simulink model "EvitaParedes23"  (R2023b)
settings: Solver=FixedStepAuto  StartTime=0.0  StopTime=inf  RelTol=1e-3  EnableMultiTasking=on
libraries: arduinolib x11, simulink x4
settings Model: PacingRate=1.500000  ExtModeTrigDuration=2  Creator=manu_  LastModifiedBy=manu_
settings OptimizationCC: EnhancedBackFolding=on  PassReuseOutputArgsAs=Individual arguments  ZeroExternalMemoryAtStartup=off  ZeroInternalMemoryAtStartup=off  MaxStackSize=64  OptimizeBlockOrder=speed  DifferentSizesBufferReuse=on  OptimizationCustomize=off  EfficientTunableParamExpr=on
settings DebuggingCC: ParameterTunabilityLossMsg=error
settings HardwareCC: ProdBitPerInt=16  ProdBitPerPointer=16  ProdBitPerSizeT=16  ProdBitPerPtrDiffT=16  ProdLargestAtomicFloat=None  ProdWordSize=8  ProdHWDeviceType=Atmel->AVR  UseEmbeddedCoderFeatures=off  UseSimulinkCoderFeatures=off
settings SFSimCC: MATLABDynamicMemAlloc=off
settings RTWCC: Description=Embedded Coder  SystemTargetFile=ert.tlc  HardwareBoard=Arduino Mega 2560  TemplateMakefile=ert_default_tmf  Toolchain=Arduino AVR  BuildConfiguration=Faster Runs
settings CodeAppCC: ForceParamTrailComments=on  IgnoreCustomStorageClasses=off  OperatorAnnotations=on  SimulinkDataObjDesc=on  SFDataObjDesc=on  MangleLength=10  InsertBlockDesc=on
settings ERTTargetCC: SupportContinuousTime=on  SupportNonInlinedSFcns=on  SupportVariableSizeSignals=on  ExtModeTransport=3  ExtModeStaticAlloc=on  ExtModeAutomaticAllocSize=off  ExtModeStaticAllocSize=2048  ExtModeMexFile=ext_xcp  ExtModeIntrfLevel=Level2 - Open

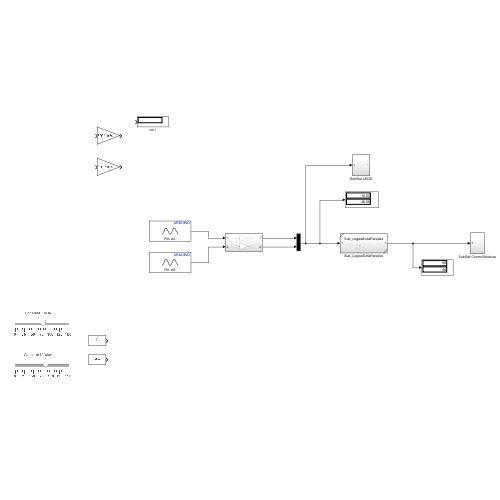
[thumbnail: Simulink's stored preview of the top-level diagram]
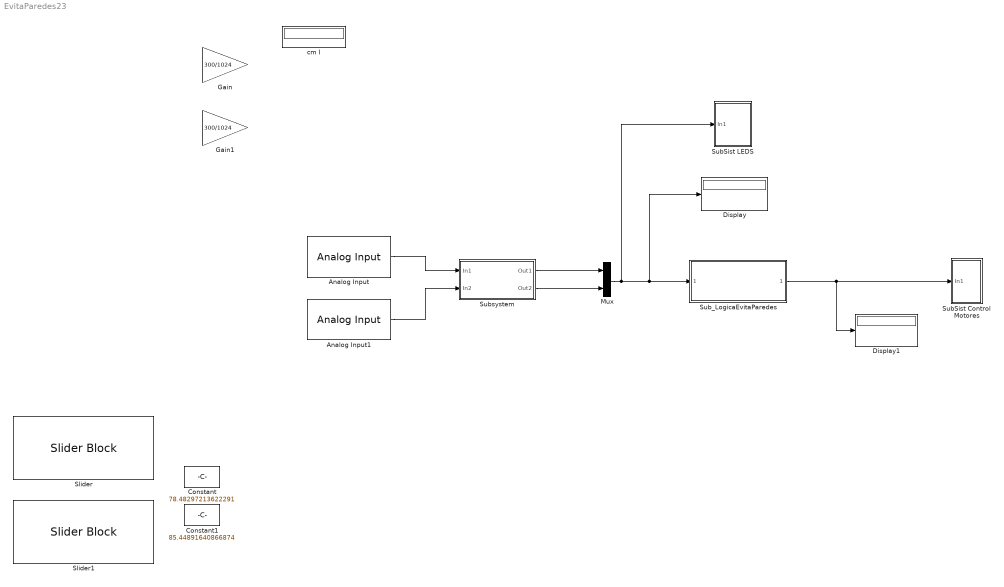
== system EvitaParedes23 ==
  Analog Input : arduinolib/Analog Input  pinNumber=4  ReadResultsOnly=off  ConversionTriggerSource=Software  ExternalTriggerType=uint32( 0 )  OutputDataType=uint16  EnableConversionCompleteNotify=off  EnableOuputStatus=off  SampleTime=-1  blockPlatform=arduino
  Analog Input1 : arduinolib/Analog Input  pinNumber=5  ReadResultsOnly=off  ConversionTriggerSource=Software  ExternalTriggerType=uint32( 0 )  OutputDataType=uint16  EnableConversionCompleteNotify=off  EnableOuputStatus=off  SampleTime=-1  blockPlatform=arduino
  Constant : Constant  Value=78.48297213622291
  Constant1 : Constant  Value=85.44891640866874
  Display : Display
  Display1 : Display
  Gain : Gain  Gain=300/1024
  Gain1 : Gain  Gain=300/1024
  Mux : Mux  Inputs=2
  Slider : SliderBlock  ScaleMax=150
  Slider1 : SliderBlock  ScaleMax=150
  SubSist Control Motores : Subsystem
  SubSist LEDS : Subsystem
  Sub_LogicaEvitaParedes : Subsystem  ReferencedSubsystem=Sub_LogicaEvitaParedes
  Subsystem : Subsystem
  cm I : Display
  wires:
  Subsystem/2(Out2) -> Mux/2
  Mux/1 -> SubSist LEDS/1(In1), Sub_LogicaEvitaParedes/1, Display/1
  Sub_LogicaEvitaParedes/1 -> SubSist Control Motores/1(In1), Display1/1
  Subsystem/1(Out1) -> Mux/1
  Analog Input/1 -> Subsystem/1(In1)
  Analog Input1/1 -> Subsystem/2(In2)

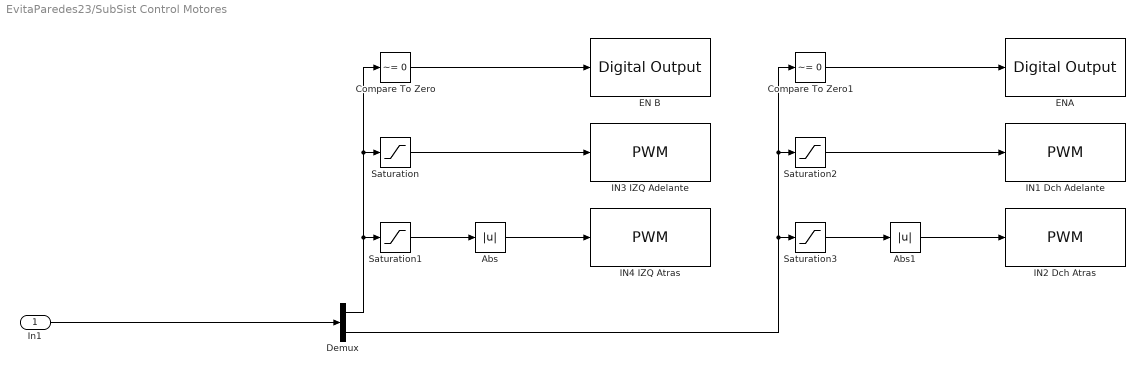
== system EvitaParedes23/SubSist Control Motores ==
  In1 : Inport
  Abs : Abs  SaturateOnIntegerOverflow=off
  Abs1 : Abs  SaturateOnIntegerOverflow=off
  Compare To Zero : simulink/Logic and Bit Operations/Compare To Zero  relop=~=  OutDataTypeStr=boolean
  Compare To Zero1 : simulink/Logic and Bit Operations/Compare To Zero  relop=~=  OutDataTypeStr=boolean
  Demux : Demux  Outputs=2
  EN B : arduinolib/Digital Output  pinNumber=13  Direction=output  blockPlatform=arduino
  ENA : arduinolib/Digital Output  pinNumber=8  Direction=output  blockPlatform=arduino
  IN1 Dch Adelante : arduinolib/PWM  pinNumber=9  frequencyType=Default  desiredFrequency=490.2  achievableFrequency=490.2
  IN2 Dch Atras : arduinolib/PWM  pinNumber=10  frequencyType=Default  desiredFrequency=490.2  achievableFrequency=490.2
  IN3 IZQ Adelante : arduinolib/PWM  pinNumber=11  frequencyType=Default  desiredFrequency=490.2  achievableFrequency=490.2
  IN4 IZQ Atras : arduinolib/PWM  pinNumber=12  frequencyType=Default  desiredFrequency=490.2  achievableFrequency=490.2
  Saturation : Saturate  UpperLimit=255  LowerLimit=0
  Saturation1 : Saturate  UpperLimit=0  LowerLimit=-255
  Saturation2 : Saturate  UpperLimit=255  LowerLimit=0
  Saturation3 : Saturate  UpperLimit=0  LowerLimit=-255
  wires:
  Demux/2 -> Compare To Zero1/1, Saturation2/1, Saturation3/1
  Demux/1 -> Compare To Zero/1, Saturation/1, Saturation1/1
  Saturation3/1 -> Abs1/1
  Compare To Zero/1 -> EN B/1
  Compare To Zero1/1 -> ENA/1
  Abs1/1 -> IN2 Dch Atras/1
  In1/1 -> Demux/1
  Abs/1 -> IN4 IZQ Atras/1
  Saturation1/1 -> Abs/1
  Saturation/1 -> IN3 IZQ Adelante/1
  Saturation2/1 -> IN1 Dch Adelante/1

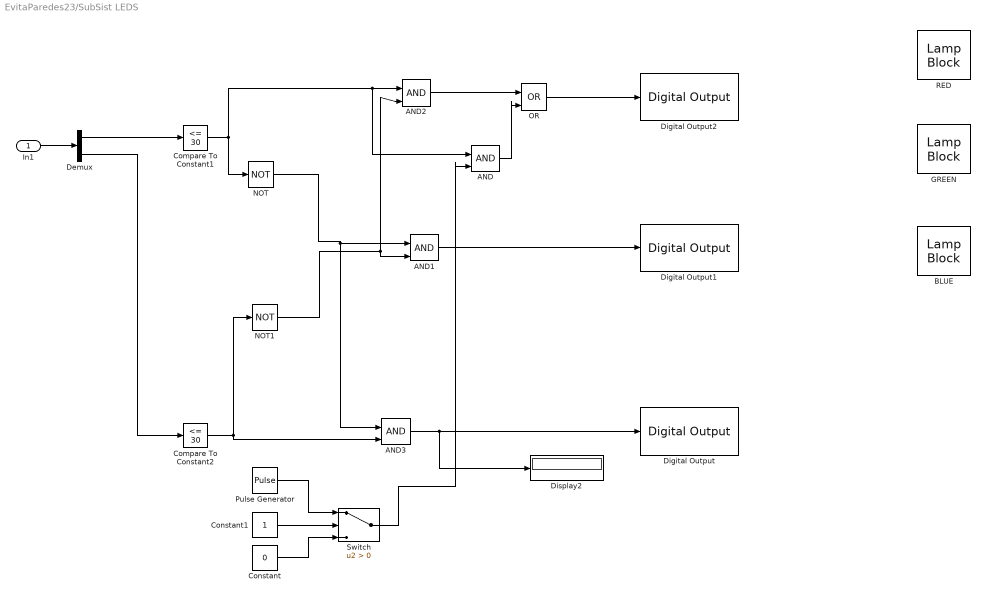
== system EvitaParedes23/SubSist LEDS ==
  In1 : Inport
  AND{,1..3} (4 alike) : Logic  IconShape=distinctive  AllPortsSameDT=off  OutDataTypeStr=boolean
  BLUE : LampBlock  LabelPosition=Hide
  Compare To Constant1 : simulink/Logic and Bit Operations/Compare To Constant  relop=<=  const=30  OutDataTypeStr=boolean
  Compare To Constant2 : simulink/Logic and Bit Operations/Compare To Constant  relop=<=  const=30  OutDataTypeStr=boolean
  Constant : Constant  Value=0
  Constant1 : Constant
  Demux : Demux  Outputs=2
  Digital Output : arduinolib/Digital Output  pinNumber=53  Direction=output  blockPlatform=arduino
  Digital Output1 : arduinolib/Digital Output  pinNumber=51  Direction=output  blockPlatform=arduino
  Digital Output2 : arduinolib/Digital Output  pinNumber=49  Direction=output  blockPlatform=arduino
  Display2 : Display
  GREEN : LampBlock  LabelPosition=Hide
  NOT : Logic  Operator=NOT  IconShape=distinctive  AllPortsSameDT=off  OutDataTypeStr=boolean
  NOT1 : Logic  Operator=NOT  IconShape=distinctive  AllPortsSameDT=off  OutDataTypeStr=boolean
  OR : Logic  Operator=OR  IconShape=distinctive  AllPortsSameDT=off  OutDataTypeStr=boolean
  Pulse Generator : DiscretePulseGenerator  PulseType=Time based  PulseWidth=50
  RED : LampBlock  LabelPosition=Hide
  Switch : Switch  Criteria=u2 > Threshold  SaturateOnIntegerOverflow=off  InputSameDT=off
  wires:
  OR/1 -> Digital Output2/1
  AND2/1 -> OR/1
  AND/1 -> OR/2
  NOT1/1 -> AND2/2, AND1/2
  Demux/2 -> Compare To Constant2/1
  NOT/1 -> AND3/1, AND1/1
  Compare To Constant2/1 -> NOT1/1, AND3/2
  In1/1 -> Demux/1
  AND3/1 -> Display2/1, Digital Output/1
  Demux/1 -> Compare To Constant1/1
  Compare To Constant1/1 -> AND/1, AND2/1, NOT/1
  AND1/1 -> Digital Output1/1
  Constant1/1 -> Switch/2
  Switch/1 -> AND/2
  Pulse Generator/1 -> Switch/1
  Constant/1 -> Switch/3

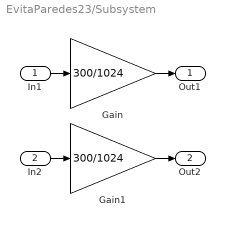
== system EvitaParedes23/Subsystem ==
  In1 : Inport
  In2 : Inport  Port=2
  Gain : Gain  Gain=300/1024
  Gain1 : Gain  Gain=300/1024
  Out1 : Outport
  Out2 : Outport  Port=2
  wires:
  In2/1 -> Gain1/1
  Gain/1 -> Out1/1
  Gain1/1 -> Out2/1
  In1/1 -> Gain/1
